simulink model "BinPicking"  (R2024b)
settings: Solver=VariableStepAuto  StartTime=0.0  StopTime=10.0  RelTol=1e-3
undefined symbols (not defined in the file): none, Sim3dSensor
libraries: robotmaniplib x2, visionstatistics x1, imaqlib x1, sim3dcameralib x1, robotsim3dlib x1, sim3dlib x1
settings Model: Creator=kiwiki  LastModifiedBy=kiwiki

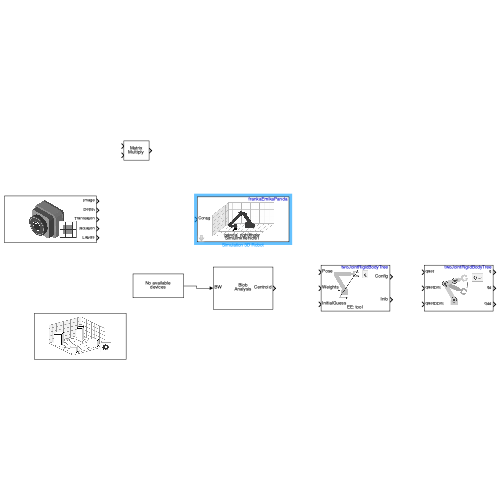
[thumbnail: Simulink's stored preview of the top-level diagram]
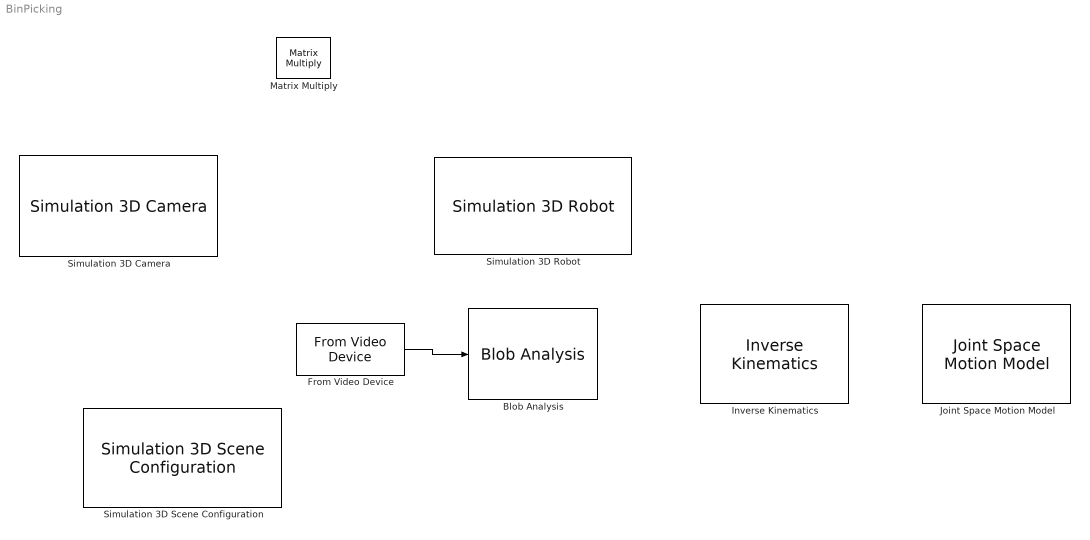
== system BinPicking ==
  Blob Analysis : visionstatistics/Blob Analysis  Tag=vipblks_row_conv  area=off  centroid=on  bBox=off  majorAxis=off  minorAxis=off  angle=off  eccentricity=off  equivDiameterSq=off  extent=off  perimeter=off  outDT=double  conn=8  isLabel=off  maxBlobs=50  warnIfNumBlobsExceeded=on  isCount=off  useMinArea=on  minArea=100  useMaxArea=off  maxArea=intmax('uint32')  excludeBorderBlob=off  isOutVarDim=off  isFill=on  fillValues=-1  roundingMode=Floor  overflowMode=off  prodOutputMode=Binary point scaling  prodOutputWordLength=32  prodOutputFracLength=16  accumMode=Binary point scaling  accumWordLength=32  accumFracLength=0  outputMode=Binary point scaling  outputWordLength=32  outputFracLength=16  firstCoeffMode=Binary point scaling  firstCoeffWordLength=16  firstCoeffFracLength=14  secondCoeffMode=Binary point scaling  secondCoeffWordLength=32  secondCoeffFracLength=16
  From Video Device : imaqlib/From Video Device  DeviceMenu=(none)  Device=(none)  ObjConstructor=(none)  VideoFormatMenu=(none)  VideoFormat=(none)  VideoSource=(none)  ROIPosition=(none)  EnableHWTrigger=off  TriggerConfiguration=none/none  SampleTime=1/30  OutputPortsMode=One multidimensional signal  DataType=single  CanDoHWTrigger=no  ReturnedColorSpace=(none)  BlockHandle=6977.0001  ROIWidth=100  ROIHeight=100  ROIColumn=0  ROIRow=0  EngXMLPath=/Applications/MATLAB_R2024b.app/toolbox/imaq/imaq/private  DevXMLPath=DEVPATH  EngLibPath=/Applications/MATLAB_R2024b.app/toolbox/imaq/imaqblks/imaqmex/maca64  ColorSpace=(none)  BayerSensorAlignment=grbg  ImaqMode=off
  Inverse Kinematics : robotmaniplib/Inverse Kinematics  RigidBodyTree=twoJointRigidBodyTree  EndEffector=tool  ShowInfo=on  SolverName=BFGS Gradient Projection  EnforceJointLimits=on  MaxIterations=1500  MaxTime=10  GradientTolerance=1e-7  SolutionTolerance=1e-6  StepTolerance=1e-14  ErrorChangeTolerance=1e-12  UseErrorDamping=on  DampingBias=0.0025  SimulateUsing=Interpreted execution
  Joint Space Motion Model : robotmaniplib/Joint Space Motion Model  RigidBodyTree=twoJointRigidBodyTree  MotionType=Computed Torque Control  ProportionalGain=100  DerivativeGain=10  ErrorDynamicsSpecification=Damping Ratio / Natural Frequency  DampingRatio=1  NaturalFrequency=10  SettlingTime=0.59  Overshoot=0  ShowExternalForcePort=off  InitConfig=0  InitJointVel=0  SimulateUsing=Interpreted execution
  Matrix Multiply : Product  Multiplication=Matrix(*)
  Simulation 3D Camera : sim3dcameralib/Simulation 3D Camera  Priority=1  sensorTag=Sim3dSensor�  sensorId=1  sensorName=Sim3dSensor�  vehTagList={'Scene Origin';'SimulinkVehicle1'}  vehTag=SimulinkVehicle1  mountLoc=Origin  offsetFlag=on  tmountOffset=[0, 0, 0]  extTmount=off  rmountOffset=[0, 0, 0]  extRmount=off  FocalLength=[1109, 1109]  OpticalCenter=[640, 360]  ImageSize=[720, 1280]  RadialDistortion=[0, 0]  TangentialDistortion=[0, 0]  SensorSkew=0  DepthOutportEnabled=on  SemanticOutportEnabled=on  TransformOutportEnabled=on  SampleTime=-1  mountPoint=[0 0 0]  mountOrientation=[0 0 0]  aMode=6  ID=1
      settings: LibrarySourceBlock=robotsim3dlib/Simulation 3D Camera
  Simulation 3D Robot : robotsim3dlib/Simulation 3D Robot  actorInputType=Robot Library  RigidBodyTree=frankaEmikaPanda  ActorName=SimulinkVehicle1  existActorChekBox=off  initialTrans=[0 0 0]  initialRot=[0 0 0]  initialConfig="[0           0           0     -1.5708           0           0           0           0           0]"  EndEffector=panda_rightfinger  eeOffsetInpChekBox=off  eeTargetTrans=[0 0 0]  eeTargetRot=[0 0 0]  enableRegionGraspChekBox=off  regionGraspInpChekBox=off  eeTargTransDiff=[0.2 0.2 0.2]  eeTargRotDiff=[0 0 0]  inpConfEnbVal=on  inpGraspEnbVal=off  inpTransEnbVal=off  outConfEnbVal=off  outGraspEnbVal=off  outTransEnbVal=off  SampleTime=0.01  ActorType=SimulinkVehicle  ID=1  aMode=6  ActorTag=SimulinkVehicle1  Mesh=RigidBodyTree
  Simulation 3D Scene Configuration : sim3dlib/Simulation 3D Scene Configuration  Priority=0  ProjectFormat=Default Scenes  SceneDesc=Empty scene  ProjectName=B:\matlab\toolbox\shared\sim3d_projects\automotive_project_windows\UE\WindowsNoEditor\VehicleSimulation.exe  ScenePath=/Game/Maps/EmptyScene  EnableOpenDRIVE=off  vehTagList={'Custom';'Scene Origin';'SimulinkVehicle1'}  vehTag=Scene Origin  FreeCameraInitialTranslation=[0, 0, 0]  FreeCameraDefaultInitialTranslation=[-6, 0, 2]  FreeCameraInitialRotation=[0, 0, 0]  FreeCameraDefaultInitialRotation=[0, -15, 0]  OpVisEn=off  Ts=0.02  EnableWindow=on  EnableRemoteAccess=off  EnableWeather=off  SunAzimuth=90  SunAltitude=40.0  EnableGeospatialSun=off  Latitude=0  Longitude=0  Date=2023-01-01  Time=10:30:00  GeoTimeZone=-5.0  SunDaylightSaving=off  wind=1  clouds=10  EnableVolumetricClouds=off  CloudCoverage=0  CloudAltitude=6  fog=0  rain=0  RaindropsEffect=off  SnowDensity=0  EnableGeospatial=off  UseTrueOrigin=off  OriginHeight=200  OriginLatitude=40.744652  OriginLongitude=-73.988864  MapStyle=Aerial  AdditionalAssetIDs=[]  UseAdvancedSunSky=off  SolarTime=11  TimeZone=-5  Day=21  Month=9  Year=2022  UseDaylightSavingTime=on  DSTStartDay=10  DSTStartMonth=3  DSTEndDay=3  DSTEndMonth=11  DSTSwitchHour=2  sensorTag=MainCamera1  sensorId=1  sensorName=MainCamera1  mountLoc=Origin  offsetFlag=off  tmountOffset=[0, 0, 0]  rmountOffset=[0, 0, 0]  HorizontalResolution=1280  VerticalResolution=720  HorizontalFOV=60  mountPoint=[0 0 0]  mountOrientation=[0 0 0]  aMode=6  ID=1  GeoTrigger=Inactive
      settings: LibrarySourceBlock=robotsim3dlib/Simulation 3D Scene Configuration
  wires:
  From Video Device/1 -> Blob Analysis/1
